simulink model "magball"  (R2021b)
settings: Solver=VariableStepAuto  StartTime=0.0  StopTime=10.0  RelTol=1e-3
settings Model: Creator=Juho  LastModifiedBy=Juho

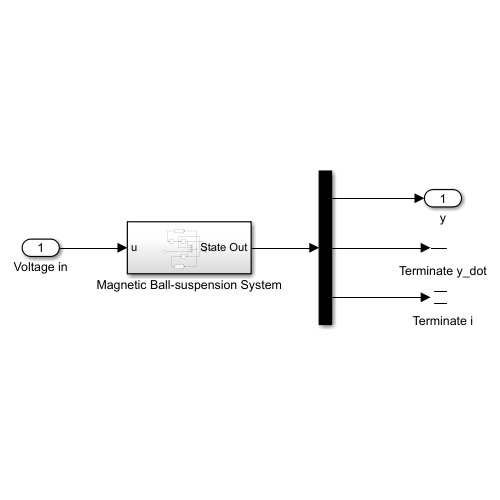
[thumbnail: Simulink's stored preview of the top-level diagram]
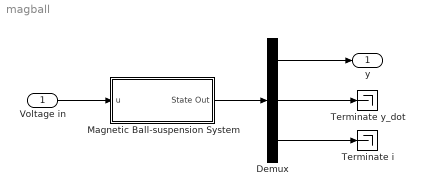
== system magball ==
  Voltage in : Inport  PortDimensions=1
  Demux : Demux  Outputs=3
  Magnetic Ball-suspension System : Subsystem
  Terminate i : Terminator
  Terminate y_dot : Terminator
  y : Outport
  wires:
  Voltage in/1 -> Magnetic Ball-suspension System/1(u)
  Magnetic Ball-suspension System/1(State Out) -> Demux/1
  Demux/3 -> Terminate i/1
  Demux/2 -> Terminate y_dot/1
  Demux/1 -> y/1

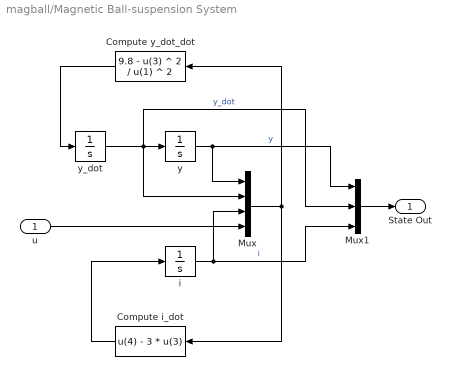
== system magball/Magnetic Ball-suspension System ==
  u : Inport
  Compute i_dot : MATLABFcn  MATLABFcn=u(4) - 3 * u(3)
  Compute y_dot_dot : MATLABFcn  MATLABFcn=9.8 - u(3) ^ 2 / u(1) ^ 2
  Mux : Mux
  Mux1 : Mux  Inputs=3
  i : Integrator
  y : Integrator
  y_dot : Integrator
  State Out : Outport
  wires:
  i/1 -> Mux/3, Mux1/3  "i"
  y_dot/1 -> Mux1/2, Mux/2, y/1  "y_dot"
  Mux/1 -> Compute i_dot/1, Compute y_dot_dot/1
  y/1 -> Mux/1, Mux1/1  "y"
  u/1 -> Mux/4
  Mux1/1 -> State Out/1
  Compute y_dot_dot/1 -> y_dot/1
  Compute i_dot/1 -> i/1
